simulink model "nn_12B"  (R2022b)
settings: Solver=VariableStepAuto  StartTime=0.0  StopTime=10.0  RelTol=1e-3
values from neighbouring files (symbols this model uses):
  b1 = [-0.578256 -0.531049 0.449559 0.391358 0.277707 0.372638 -0.130073 0.423662 0.414256 -0.378106]    [new_nn_12B_data.mat]
  b2 = [-0.561938 -0.812212 -0.549473 -0.549797 -1.080223 0.652062 0.234581 1.306192 2.051893 -0.89138]    [new_nn_12B_data.mat]
  b3 = -0.01575    [new_nn_12B_data.mat]
  Hecate_RangeX = 0.0381947846056    [new_nn_12B_data.mat]
  meaninp = [-0.014928 -0.08076]    [new_nn_12B_data.mat]
  meanout = -0.01416    [new_nn_12B_data.mat]
  oostdinp = [0.918012 0.847388]    [new_nn_12B_data.mat]
  stdevout = 0.205    [new_nn_12B_data.mat]
  w1 = [-0.65101 1.000785 -0.225403 -1.250849 0.006928 0.402083 -0.27538 -0.375693 -0.343296 -0.963722 0.413488 0.166138 ... (20 elements, 2x10)]    [new_nn_12B_data.mat]
  w2 = [-0.059798 -0.128454 -0.107191 0.724165 -0.291639 -0.929753 -0.379182 0.996259 -0.416213 0.884865 -0.710416 -0.421403 ... (100 elements, 10x10)]    [new_nn_12B_data.mat]
  w3 = [-0.482061 0.739126 0.886125 1.875287 -0.959398 1.77256 -0.303801 0.909694 -0.681003 -0.930787]    [new_nn_12B_data.mat]
  xinmax = [1.885733 1.974943]    [new_nn_12B_data.mat]
  xinmin = [-1.969179 -1.999644]    [new_nn_12B_data.mat]
undefined symbols (not defined in the file or in its folder): Hecate_RangeX2, Hecate_RangeY, Hecate_RangeY2
(part 2 of 2)

== system nn_12B/nn_2x10x10x1/Neuron Layer 2/Neuron 7/If Action Subsystem3 ==
  In1 : Inport
  Action Port : ActionPort  ActionPortLabel=else
  Sum : Sum  Inputs=|++
  bias1 : Constant  Value=0.990025
  weight1 : Gain  Gain=0.01
  Out1 : Outport
  wires:
  bias1/1 -> Sum/2
  weight1/1 -> Sum/1
  In1/1 -> weight1/1
  Sum/1 -> Out1/1

== system nn_12B/nn_2x10x10x1/Neuron Layer 2/Neuron 8/If Action Subsystem ==
  In1 : Inport
  Action Port : ActionPort  ActionPortLabel=if(u1 < -0.995)
  Sum : Sum  Inputs=|+-
  bias1 : Constant  Value=0.990025
  weight1 : Gain  Gain=0.01
  Out1 : Outport
  wires:
  bias1/1 -> Sum/2
  weight1/1 -> Sum/1
  In1/1 -> weight1/1
  Sum/1 -> Out1/1

== system nn_12B/nn_2x10x10x1/Neuron Layer 2/Neuron 8/If Action Subsystem1 ==
  In1 : Inport
  Action Port : ActionPort  ActionPortLabel=elseif(u1 < 0)
  Product1 : Product  RndMeth=Zero
  Sum3 : Sum  Inputs=|++
  bias4 : Constant  Value=2
  Out1 : Outport
  wires:
  In1/1 -> Product1/1, Sum3/1
  bias4/1 -> Sum3/2
  Sum3/1 -> Product1/2
  Product1/1 -> Out1/1

== system nn_12B/nn_2x10x10x1/Neuron Layer 2/Neuron 8/If Action Subsystem2 ==
  In1 : Inport
  Action Port : ActionPort  ActionPortLabel=elseif( u1<0.995)
  Product1 : Product  RndMeth=Zero
  Sum3 : Sum  Inputs=|-+
  bias4 : Constant  Value=2
  Out1 : Outport
  wires:
  Product1/1 -> Out1/1
  Sum3/1 -> Product1/2
  bias4/1 -> Sum3/2
  In1/1 -> Sum3/1, Product1/1

== system nn_12B/nn_2x10x10x1/Neuron Layer 2/Neuron 8/If Action Subsystem3 ==
  In1 : Inport
  Action Port : ActionPort  ActionPortLabel=else
  Sum : Sum  Inputs=|++
  bias1 : Constant  Value=0.990025
  weight1 : Gain  Gain=0.01
  Out1 : Outport
  wires:
  bias1/1 -> Sum/2
  weight1/1 -> Sum/1
  In1/1 -> weight1/1
  Sum/1 -> Out1/1

== system nn_12B/nn_2x10x10x1/Neuron Layer 2/Neuron 9/If Action Subsystem ==
  In1 : Inport
  Action Port : ActionPort  ActionPortLabel=if(u1 < -0.995)
  Sum : Sum  Inputs=|+-
  bias1 : Constant  Value=0.990025
  weight1 : Gain  Gain=0.01
  Out1 : Outport
  wires:
  bias1/1 -> Sum/2
  weight1/1 -> Sum/1
  In1/1 -> weight1/1
  Sum/1 -> Out1/1

== system nn_12B/nn_2x10x10x1/Neuron Layer 2/Neuron 9/If Action Subsystem1 ==
  In1 : Inport
  Action Port : ActionPort  ActionPortLabel=elseif(u1 < 0)
  Product1 : Product  RndMeth=Zero
  Sum3 : Sum  Inputs=|++
  bias4 : Constant  Value=2
  Out1 : Outport
  wires:
  In1/1 -> Product1/1, Sum3/1
  bias4/1 -> Sum3/2
  Sum3/1 -> Product1/2
  Product1/1 -> Out1/1

== system nn_12B/nn_2x10x10x1/Neuron Layer 2/Neuron 9/If Action Subsystem2 ==
  In1 : Inport
  Action Port : ActionPort  ActionPortLabel=elseif( u1<0.995)
  Product1 : Product  RndMeth=Zero
  Sum3 : Sum  Inputs=|-+
  bias4 : Constant  Value=2
  Out1 : Outport
  wires:
  Product1/1 -> Out1/1
  Sum3/1 -> Product1/2
  bias4/1 -> Sum3/2
  In1/1 -> Sum3/1, Product1/1

== system nn_12B/nn_2x10x10x1/Neuron Layer 2/Neuron 9/If Action Subsystem3 ==
  In1 : Inport
  Action Port : ActionPort  ActionPortLabel=else
  Sum : Sum  Inputs=|++
  bias1 : Constant  Value=0.990025
  weight1 : Gain  Gain=0.01
  Out1 : Outport
  wires:
  bias1/1 -> Sum/2
  weight1/1 -> Sum/1
  In1/1 -> weight1/1
  Sum/1 -> Out1/1

== stateflow chart nn_12B/Test Assessment ==
  state step_1
    verify(z <= 1.1 && z >= -0.2)
  (default) -> step_1
  data: z input

== stateflow chart nn_12B/Test Sequence ==
  state step_1
    x = 0+Hecate_RangeX;
    y = 0+Hecate_RangeY;
  state step_2
    x = 0+Hecate_RangeX2;
    y = 0+Hecate_RangeY2;
  (default) -> step_1
  step_1 -> step_2 : [
      | after(50,sec)
      | ]
  data: x output; y output; Hecate_RangeX parameter; Hecate_RangeY parameter; Hecate_RangeX2 parameter; Hecate_RangeY2 parameter
